simulink model "Test1_DSRC_Vs_CV2X"  (R2024b)
settings: Solver=VariableStepAuto  StartTime=0.0  StopTime=10  RelTol=1e-3
undefined symbols (not defined in the file): dataRate_CV2X, dataRate_DSRC, lossRate_CV2X, lossRate_DSRC, numPackets, packetSize
libraries: simulink x4

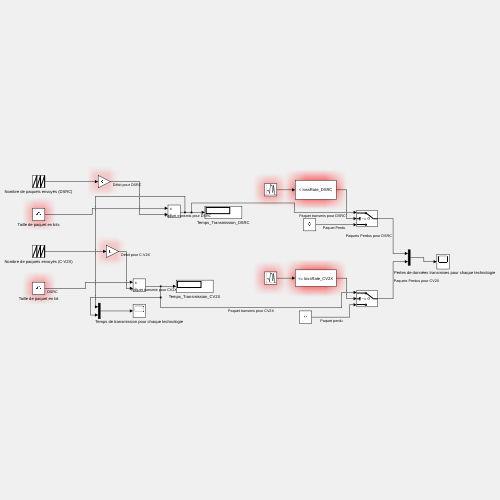
[thumbnail: Simulink's stored preview of the top-level diagram]
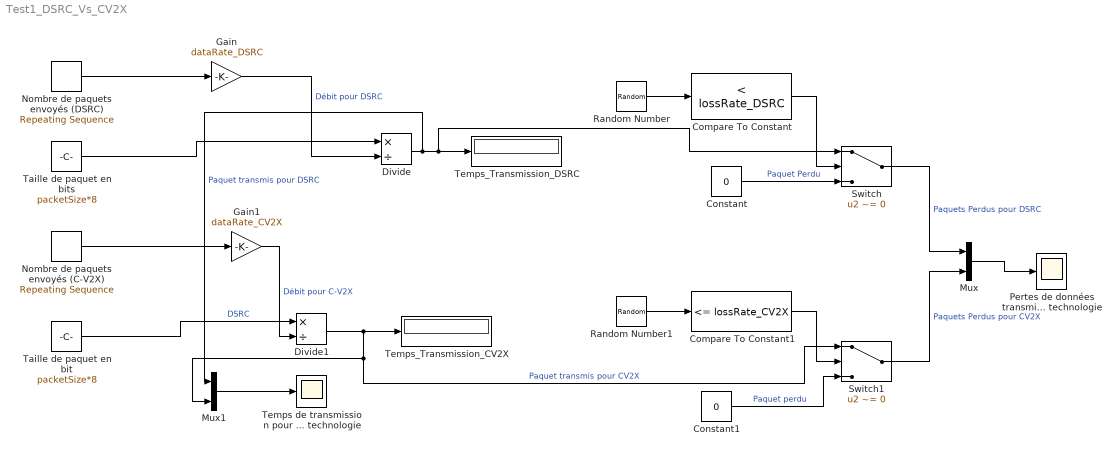
== system Test1_DSRC_Vs_CV2X ==
  "   Pertes de données transmises pour chaque technologie" : Scope
  Compare To Constant : simulink/Logic and Bit Operations/Compare To Constant  relop=<  const=lossRate_DSRC  OutDataTypeStr=boolean
  Compare To Constant1 : simulink/Logic and Bit Operations/Compare To Constant  relop=<=  const=lossRate_CV2X  OutDataTypeStr=boolean
  Constant : Constant  Value=0
  Constant1 : Constant  Value=0
  Divide : Product  Inputs=*/
  Divide1 : Product  Inputs=*/
  Gain : Gain  Gain=dataRate_DSRC
  Gain1 : Gain  Gain=dataRate_CV2X
  Mux : Mux  Inputs=2
  Mux1 : Mux  Inputs=2
  Nombre de paquets envoyés (C-V2X) : simulink/Sources/Repeating Sequence  rep_seq_t=[0 10000]  rep_seq_y=[0 10000]
  Nombre de paquets envoyés (DSRC) : simulink/Sources/Repeating Sequence  rep_seq_t=[0 10000]  rep_seq_y=[0 10000]
  Random Number : RandomNumber  Variance=numPackets  SampleTime=0.1
  Random Number1 : RandomNumber  Variance=numPackets  SampleTime=0.1
  Switch : Switch  Criteria=u2 ~= 0  SaturateOnIntegerOverflow=off  InputSameDT=off
  Switch1 : Switch  Criteria=u2 ~= 0  SaturateOnIntegerOverflow=off  InputSameDT=off
  Taille de paquet en bit : Constant  Value=packetSize*8
  Taille de paquet en bits : Constant  Value=packetSize*8
  Temps de transmission pour chaque technologie : Scope
  Temps_Transmission_CV2X : Display
  Temps_Transmission_DSRC : Display
  wires:
  Divide/1 -> Mux1/1, Switch/1, Temps_Transmission_DSRC/1  "Paquet transmis pour DSRC"
  Divide1/1 -> Mux1/2, Switch1/1, Temps_Transmission_CV2X/1  "Paquet transmis pour CV2X"
  Nombre de paquets envoyés (DSRC)/1 -> Gain/1
  Nombre de paquets envoyés (C-V2X)/1 -> Gain1/1
  Gain/1 -> Divide/2  "Débit pour DSRC"
  Taille de paquet en bits/1 -> Divide/1
  Gain1/1 -> Divide1/2  "Débit pour C-V2X"
  Taille de paquet en bit/1 -> Divide1/1  "DSRC"
  Random Number/1 -> Compare To Constant/1
  Random Number1/1 -> Compare To Constant1/1
  Compare To Constant/1 -> Switch/2
  Constant/1 -> Switch/3  "Paquet Perdu"
  Compare To Constant1/1 -> Switch1/2
  Constant1/1 -> Switch1/3  "Paquet perdu"
  Switch/1 -> Mux/1  "Paquets Perdus pour DSRC"
  Switch1/1 -> Mux/2  "Paquets Perdus pour CV2X"
  Mux/1 -> "   Pertes de données transmises pour chaque technologie"/1
  Mux1/1 -> Temps de transmission pour chaque technologie/1
